simulink model "CAT797_lateral_dynamics_open_loop_SMC"  (R2026a)
settings: Solver=ode4  StopTime=40  FixedStep=0.0001
undefined symbols (not defined in the file): Cf, Cr, ktan, lambda, lambda2, Lf, Lr, nutan
libraries: simulink_extras x1, lat_dyn_haul_00 x1
settings Model: DataDictionary=CAT_797F.sldd  Creator=Local1  LastModifiedBy=Local1
settings DebuggingCC: InheritedTsInSrcMsg=none

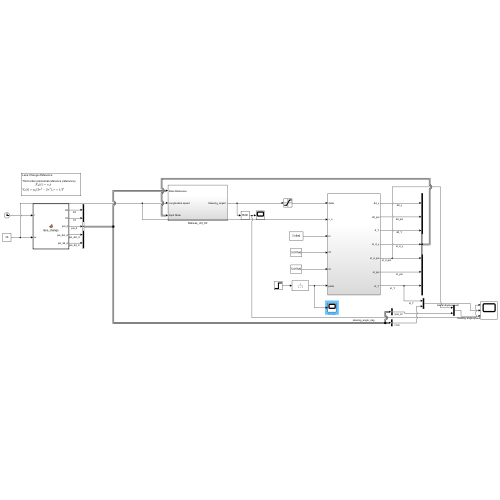
[thumbnail: Simulink's stored preview of the top-level diagram]
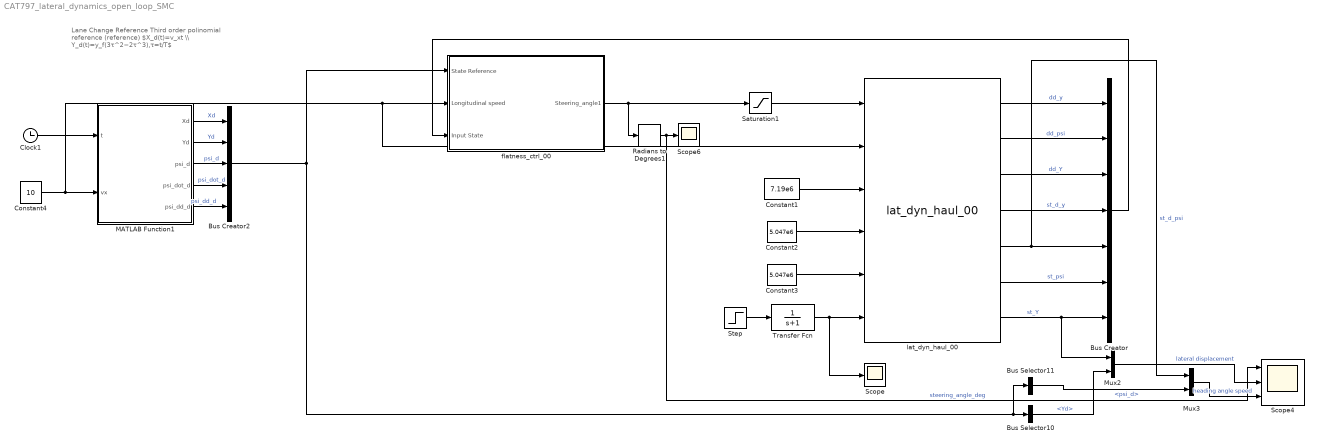
== system CAT797_lateral_dynamics_open_loop_SMC ==
  note: Lane Change Reference
      |
      | Third order polinomial reference (reference)
      | $X_d​(t)=v_x​t \\ Y_d(t)=y_f(3τ^2−2τ^3),τ=t/T$
  Bus Creator : BusCreator  Inputs=7
  Bus Creator2 : BusCreator  Inputs=5
  Bus Selector10 : BusSelector  OutputSignals=Yd
  Bus Selector11 : BusSelector  OutputSignals=psi_d
  Clock1 : Clock
  Constant1 : Constant  Value=7.19e6
  Constant2 : Constant  Value=5.047e6
  Constant3 : Constant  Value=5.047e6
  Constant4 : Constant  Value=10
  MATLAB Function1 : MATLAB Function  TreatAsAtomicUnit=on
  Mux2 : Mux  Inputs=2
  Mux3 : Mux  Inputs=2
  Radians to Degrees1 : simulink_extras/Transformations/Radians to Degrees
  Saturation1 : Saturate  UpperLimit=25  LowerLimit=-25
  Scope : Scope
      settings: ActiveDisplayYMinimum=-0.124999994825164  ActiveDisplayYMaximum=1.1249999534264763
  Scope4 : Scope  NumInputPorts=3
      settings: ActiveDisplayString=3  ActiveDisplayYMinimum=-0.091602834580546313  ActiveDisplayYMaximum=0.068955881009726411  DataLoggingVariableName=ScopeData7
  Scope6 : Scope
      settings: ActiveDisplayYMinimum=-1  ActiveDisplayYMaximum=1  DataLoggingVariableName=ScopeData9
  Step : Step  Time=23  SampleTime=0
  Transfer Fcn : TransferFcn  Denominator=[1 1]
  flatness_ctrl_00 : Subsystem
  lat_dyn_haul_00 : lat_dyn_haul_00/lat_dyn_haul_00  SystemSampleTime=-1  VariantActivationTime=update diagram  EmptyChoice=off  PassThrough=off  PassThroughVariantControl=(default)  EmptyChoiceVariantControl=(default)  AllowFlexibleInterface=on  Latency=0  AutoFrameSizeCalculation=off
      link override Subsystem/Integrator1: InitialCondition=0.01
  wires:
  MATLAB Function1/4(psi_dot_d) -> Bus Creator2/4  "psi_dot_d"
  Bus Creator2/1 -> flatness_ctrl_00/1(State Reference), Bus Selector11/1, Bus Selector10/1
  Mux2/1 -> Scope4/2  "lateral displacement"
  lat_dyn_haul_00/6 -> Bus Creator/6  "st_psi"
  Bus Creator/1 -> flatness_ctrl_00/3(Input State)
  Constant1/1 -> lat_dyn_haul_00/3
  lat_dyn_haul_00/7 -> Mux2/1, Bus Creator/7  "st_Y"
  MATLAB Function1/5(psi_dd_d) -> Bus Creator2/5  "psi_dd_d"
  Constant3/1 -> lat_dyn_haul_00/5
  MATLAB Function1/3(psi_d) -> Bus Creator2/3  "psi_d"
  Mux3/1 -> Scope4/3  "heading angle speed"
  Saturation1/1 -> lat_dyn_haul_00/1
  Radians to Degrees1/1 -> Scope4/1, Scope6/1  "steering_angle_deg"
  Clock1/1 -> MATLAB Function1/1(t)
  Constant4/1 -> lat_dyn_haul_00/2, flatness_ctrl_00/2(Longitudinal speed), MATLAB Function1/2(vx)
  Bus Selector10/1 -> Mux2/2  "<Yd>"
  lat_dyn_haul_00/1 -> Bus Creator/1  "dd_y"
  lat_dyn_haul_00/4 -> Bus Creator/4  "st_d_y"
  MATLAB Function1/1(Xd) -> Bus Creator2/1  "Xd"
  MATLAB Function1/2(Yd) -> Bus Creator2/2  "Yd"
  flatness_ctrl_00/1(Steering_angle1) -> Radians to Degrees1/1, Saturation1/1
  lat_dyn_haul_00/3 -> Bus Creator/3  "dd_Y"
  Constant2/1 -> lat_dyn_haul_00/4
  Bus Selector11/1 -> Mux3/2  "<psi_d>"
  lat_dyn_haul_00/5 -> Mux3/1, Bus Creator/5  "st_d_psi"
  lat_dyn_haul_00/2 -> Bus Creator/2  "dd_psi"
  Step/1 -> Transfer Fcn/1
  Transfer Fcn/1 -> Scope/1, lat_dyn_haul_00/6

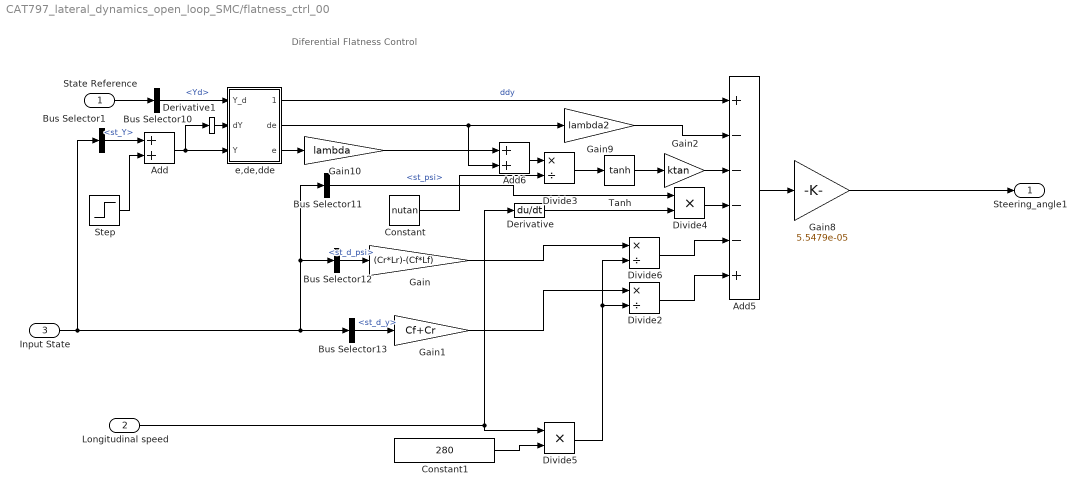
== system CAT797_lateral_dynamics_open_loop_SMC/flatness_ctrl_00 ==
  note: Diferential Flatness Control
  State Reference : Inport
  Longitudinal speed : Inport  Port=2
  Input State : Inport  Port=3
  Add : Sum
  Add5 : Sum  Inputs=+----+
  Add6 : Sum
  Bus Selector1 : BusSelector  OutputSignals=st_Y
  Bus Selector10 : BusSelector  OutputSignals=Yd
  Bus Selector11 : BusSelector  OutputSignals=st_psi
  Bus Selector12 : BusSelector  OutputSignals=st_d_psi
  Bus Selector13 : BusSelector  OutputSignals=st_d_y
  Constant : Constant  Value=nutan
  Constant1 : Constant  Value=280
  Derivative : Derivative
  Derivative1 : Derivative
  Divide2 : Product  Inputs=*/
  Divide3 : Product  Inputs=*/
  Divide4 : Product  Inputs=**
  Divide5 : Product  Inputs=**
  Divide6 : Product  Inputs=*/
  Gain : Gain  Gain=(Cr*Lr)-(Cf*Lf)
  Gain1 : Gain  Gain=Cf+Cr
  Gain10 : Gain  Gain=lambda
  Gain2 : Gain  Gain=ktan
  Gain8 : Gain  Gain=5.5479e-05  OutDataTypeStr=double
  Gain9 : Gain  Gain=lambda2
  Step : Step  Time=20  FinalValue=0  SampleTime=0
  Tanh : Trigonometry  Operator=tanh
  e,de,dde : Subsystem
  Steering_angle1 : Outport
  wires:
  Input State/1 -> Bus Selector13/1, Bus Selector11/1, Bus Selector12/1, Bus Selector1/1
  State Reference/1 -> Bus Selector10/1
  Longitudinal speed/1 -> Derivative/1, Divide5/1
  Bus Selector10/1 -> e,de,dde/1(Y_d)  "<Yd>"
  Gain8/1 -> Steering_angle1/1
  Add5/1 -> Gain8/1
  e,de,dde/1(ddY_d) -> Add5/1  "ddy"
  Gain9/1 -> Add5/2
  e,de,dde/2(de) -> Add6/2, Gain9/1
  e,de,dde/3(e) -> Gain10/1
  Gain10/1 -> Add6/1
  Add6/1 -> Divide3/1
  Constant/1 -> Divide3/2
  Divide3/1 -> Tanh/1
  Bus Selector11/1 -> Divide4/1  "<st_psi>"
  Derivative/1 -> Divide4/2
  Divide4/1 -> Add5/4
  Constant1/1 -> Divide5/2
  Divide5/1 -> Divide2/2, Divide6/2
  Divide6/1 -> Add5/5
  Bus Selector12/1 -> Gain/1  "<st_d_psi>"
  Gain/1 -> Divide6/1
  Divide2/1 -> Add5/6
  Bus Selector13/1 -> Gain1/1  "<st_d_y>"
  Gain1/1 -> Divide2/1
  Derivative1/1 -> e,de,dde/2(dY)
  Gain2/1 -> Add5/3
  Tanh/1 -> Gain2/1
  Bus Selector1/1 -> Add/1  "<st_Y>"
  Add/1 -> e,de,dde/3(Y), Derivative1/1
  Step/1 -> Add/2

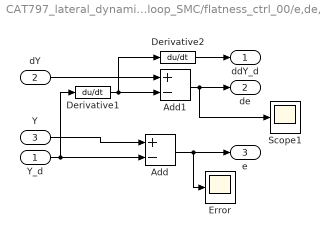
== system CAT797_lateral_dynamics_open_loop_SMC/flatness_ctrl_00/e,de,dde ==
  Y_d : Inport
  dY : Inport  Port=2
  Y : Inport  Port=3
  Add : Sum  Inputs=+-
  Add1 : Sum  Inputs=+-
  Derivative1 : Derivative
  Derivative2 : Derivative
  Error : Scope
      settings: ActiveDisplayYMinimum=-1.2059525791827523  ActiveDisplayYMaximum=0.59595586586598426  DataLoggingVariableName=ScopeData2
  Scope1 : Scope
      settings: ActiveDisplayYMinimum=-1290.5420882367673  ActiveDisplayYMaximum=11159.763925727051  DataLoggingVariableName=ScopeData3
  ddY_d : Outport
  de : Outport  Port=2
  e : Outport  Port=3
  wires:
  Add/1 -> e/1, Error/1
  Y/1 -> Add/1
  Derivative1/1 -> Derivative2/1, Add1/2
  Derivative2/1 -> ddY_d/1
  Y_d/1 -> Derivative1/1, Add/2
  Add1/1 -> Scope1/1, de/1
  dY/1 -> Add1/1

== matlab function CAT797_lateral_dynamics_open_loop_SMC/MATLAB Function1 ==
  data: t input; Xd output; vx input; Yd output; psi_d output; psi_dot_d output; psi_dd_d output
function [Xd, Yd, psi_d, psi_dot_d, psi_dd_d] = lane_change(t, vx)

% PARAMETERS (tune these)
T  = 10;       % duration [s]
yf = 3.5;      % lateral shift [m]

% Normalize time
tau = t / T;

% Clamp tau between 0 and 1
if tau > 1
    tau = 1;
end
if tau < 0
    tau = 0;
end

% =========================
% POSITION
% =========================
Xd = vx * t;
Yd = yf * (3*tau^2 - 2*tau^3);

% =========================
% FIRST DERIVATIVE
% =========================
Xd_dot = vx;
Yd_dot = yf * (6*tau/T - 6*tau^2/T);

% =========================
% SECOND DERIVATIVE
% =========================
Xd_ddot = 0;
Yd_ddot = yf * (6/T^2 - 12*tau/T^2);

% =========================
% HEADING
% =========================
psi_d = atan2(Yd_dot, Xd_dot);

% =========================
% YAW RATE
% =========================
psi_dot_d = (Xd_dot * Yd_ddot - Yd_dot * Xd_ddot) / ...
            (Xd_dot^2 + Yd_dot^2);

% =========================
% YAW ACCELERATION (optional)
% =========================
% Numerical approximation (simple)
dt = 1e-3;

tau2 = (t+dt)/T;
if tau2 > 1
    tau2 = 1;
end

Yd_dot_2 = yf * (6*tau2/T - 6*tau2^2/T);
psi_d_2 = atan2(Yd_dot_2, vx);

psi_dd_d = (psi_d_2 - psi_d) / dt;

end
